simulink model "button"  (R2021b)
settings: Solver=FixedStepDiscrete  StartTime=0.0  StopTime=inf  FixedStep=0.01  RelTol=1e-3
libraries: robotlib x11, simulink x2
settings Model: Creator=alessandrini  LastModifiedBy=alessandrini
settings OptimizationCC: EnhancedBackFolding=on  PassReuseOutputArgsAs=Individual arguments  ZeroExternalMemoryAtStartup=off  ZeroInternalMemoryAtStartup=off  MaxStackSize=64  OptimizeBlockOrder=speed  DifferentSizesBufferReuse=on  OptimizationCustomize=off  EfficientTunableParamExpr=on
settings DebuggingCC: ParameterTunabilityLossMsg=error
settings HardwareCC: ProdBitPerPointer=32  ProdBitPerSizeT=32  ProdBitPerPtrDiffT=32  ProdLargestAtomicFloat=None  ProdIntDivRoundTo=Undefined  ProdEndianess=Unspecified  ProdWordSize=32  ProdHWDeviceType=Generic->Unspecified (assume 32-bit Generic)  UseEmbeddedCoderFeatures=off
settings RTWCC: Description=Embedded Coder  SystemTargetFile=ert.tlc  HardwareBoard=Robot Operating System (ROS)  TLCOptions="-aInlineSetEventsForThisBaseRateFcn=TLC_FALSE -aSuppressMultiTaskScheduler=TLC_FALSE  -aRateBasedStepFcn=0"  TemplateMakefile=ert_default_tmf  Toolchain=Catkin  TargetLang=C++
settings CodeAppCC: ForceParamTrailComments=on  IgnoreCustomStorageClasses=off  OperatorAnnotations=on  SimulinkDataObjDesc=on  SFDataObjDesc=on  InsertBlockDesc=on
settings ERTTargetCC: SupportNonInlinedSFcns=on

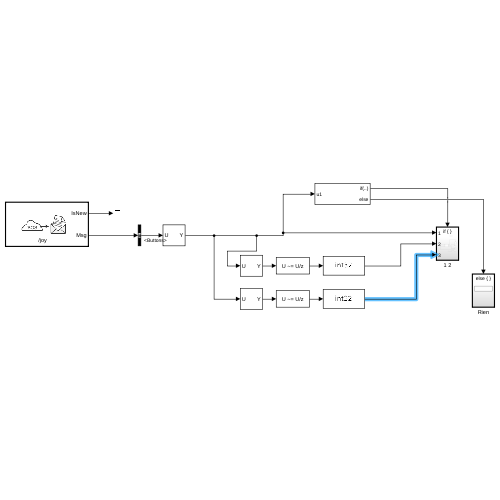
[thumbnail: Simulink's stored preview of the top-level diagram]
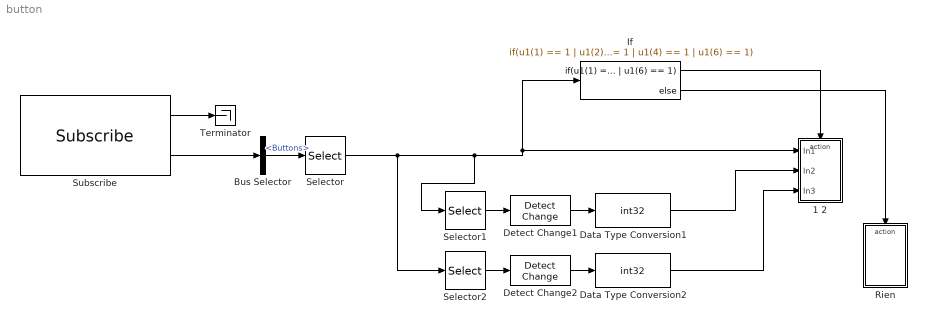
== system button ==
  1 2 : Subsystem
  Bus Selector : BusSelector  OutputSignals=Buttons
  Data Type Conversion1 : DataTypeConversion  OutDataTypeStr=int32
  Data Type Conversion2 : DataTypeConversion  OutDataTypeStr=int32
  Detect Change1 : simulink/Logic and Bit Operations/Detect Change  vinit=0  OutDataTypeStr=boolean
  Detect Change2 : simulink/Logic and Bit Operations/Detect Change  vinit=0  OutDataTypeStr=boolean
  If : If  IfExpression=u1(1) == 1 | u1(2) == 1 | u1(3) == 1 | u1(4) == 1 | u1(6) == 1
  Rien : Subsystem
  Selector : Selector  InputPortWidth=128  IndexOptions=Index vector (dialog)  Indices=[1 2 3 4 5 6]  OutputSizes=1
  Selector1 : Selector  InputPortWidth=6  IndexOptions=Index vector (dialog)  Indices=[1]  OutputSizes=1
  Selector2 : Selector  InputPortWidth=6  IndexOptions=Index vector (dialog)  Indices=[3]  OutputSizes=1
  Subscribe : robotlib/Subscribe  topicSource=Select from ROS network  topic=/joy  messageType=sensor_msgs/Joy  SampleTime=-1  legacyBusStruct=off  messageQueueLength=1
  Terminator : Terminator
  wires:
  Subscribe/2 -> Bus Selector/1
  Subscribe/1 -> Terminator/1
  If/2 -> Rien/Action
  If/1 -> 1 2/Action
  Bus Selector/1 -> Selector/1  "<Buttons>"
  Selector/1 -> Selector2/1, Selector1/1, If/1, 1 2/1(In1)
  Detect Change1/1 -> Data Type Conversion1/1
  Data Type Conversion1/1 -> 1 2/2(In2)
  Selector1/1 -> Detect Change1/1
  Selector2/1 -> Detect Change2/1
  Detect Change2/1 -> Data Type Conversion2/1
  Data Type Conversion2/1 -> 1 2/3(In3)

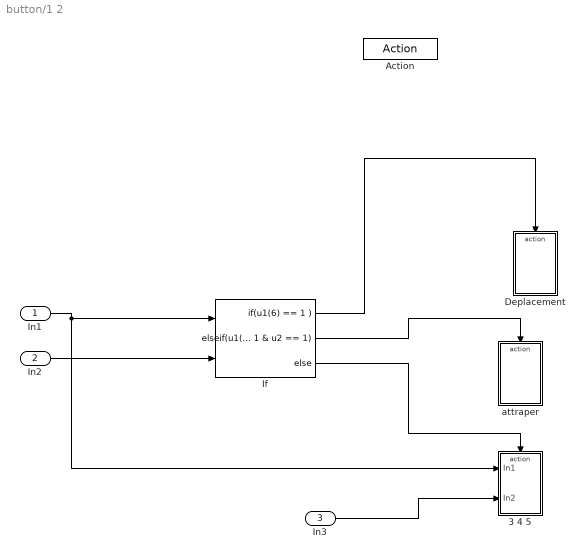
== system button/1 2 ==
  In1 : Inport
  In2 : Inport  Port=2
  In3 : Inport  Port=3
  Action : ActionPort  InitializeStates=reset  ActionPortLabel=if(u1(1) == 1 | u1(2) == 1 | u1(3) == 1 | u1(4) == 1 | u1(6) == 1)
  3 4 5 : Subsystem
  Deplacement : Subsystem
  If : If  NumInputs=2  IfExpression=u1(6) == 1  ElseIfExpressions=u1(1) == 1 & u2 == 1
  attraper : Subsystem
  wires:
  In1/1 -> 3 4 5/1(In1), If/1
  If/1 -> Deplacement/Action
  If/2 -> attraper/Action
  If/3 -> 3 4 5/Action
  In2/1 -> If/2
  In3/1 -> 3 4 5/2(In2)

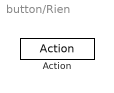
== system button/Rien ==
  Action : ActionPort  InitializeStates=reset  ActionPortLabel=else

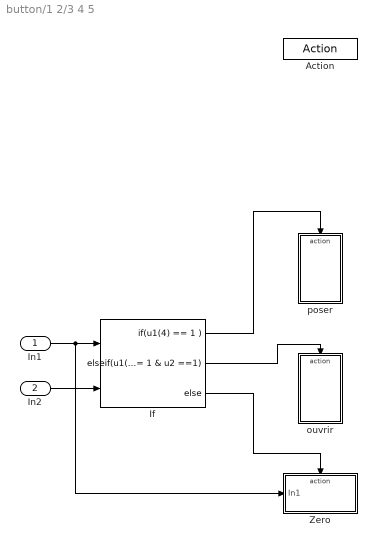
== system button/1 2/3 4 5 ==
  In1 : Inport
  In2 : Inport  Port=2
  Action : ActionPort  InitializeStates=reset  ActionPortLabel=else
  If : If  NumInputs=2  IfExpression=u1(4) == 1  ElseIfExpressions=u1(3) == 1 & u2 ==1
  "Zero " : Subsystem  TreatAsAtomicUnit=on
  ouvrir : Subsystem
  poser : Subsystem
  wires:
  If/3 -> "Zero "/Action
  If/2 -> ouvrir/Action
  In1/1 -> "Zero "/1(In1), If/1
  If/1 -> poser/Action
  In2/1 -> If/2

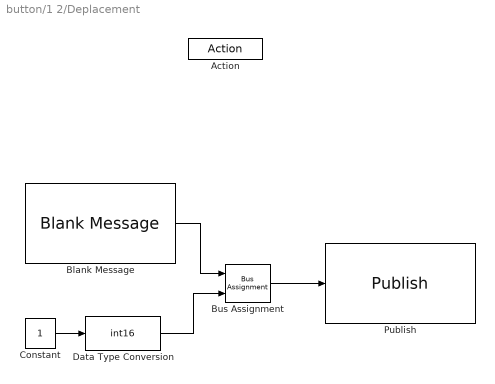
== system button/1 2/Deplacement ==
  Action : ActionPort  InitializeStates=reset  ActionPortLabel=if(u1(6) == 1 )
  Blank Message : robotlib/Blank Message  messageClass=Message  entityType=std_msgs/Int16  messageType=std_msgs/Int16  SampleTime=inf  legacyBusStruct=off
  Bus Assignment : BusAssignment  AssignedSignals=Data
  Constant : Constant
  Data Type Conversion : DataTypeConversion  OutDataTypeStr=int16
  Publish : robotlib/Publish  topicSource=Specify your own  topic=/etat  messageType=std_msgs/Int16  legacyBusStruct=off  messageQueueLength=1
  wires:
  Blank Message/1 -> Bus Assignment/1
  Bus Assignment/1 -> Publish/1
  Constant/1 -> Data Type Conversion/1
  Data Type Conversion/1 -> Bus Assignment/2
  ? -> ?
  ? -> ?

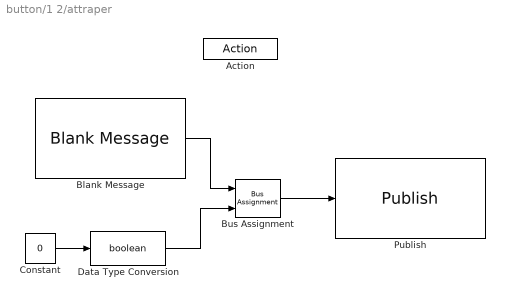
== system button/1 2/attraper ==
  Action : ActionPort  InitializeStates=reset  ActionPortLabel=elseif(u1(1) == 1 )
  Blank Message : robotlib/Blank Message  messageClass=Message  entityType=std_msgs/Bool  messageType=std_msgs/Bool  SampleTime=inf  legacyBusStruct=off
  Bus Assignment : BusAssignment  AssignedSignals=Data
  Constant : Constant  Value=0
  Data Type Conversion : DataTypeConversion  OutDataTypeStr=boolean
  Publish : robotlib/Publish  topicSource=Specify your own  topic=/hand  messageType=std_msgs/Bool  legacyBusStruct=off  messageQueueLength=1
  wires:
  Data Type Conversion/1 -> Bus Assignment/2
  Bus Assignment/1 -> Publish/1
  Constant/1 -> Data Type Conversion/1
  Blank Message/1 -> Bus Assignment/1

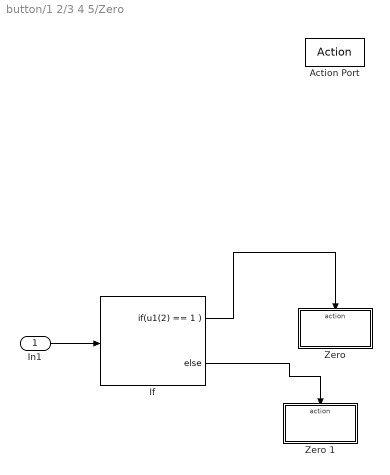
== system button/1 2/3 4 5/Zero  ==
  In1 : Inport
  Action Port : ActionPort  ActionPortLabel=else
  If : If  IfExpression=u1(2) == 1
  "Zero " : Subsystem  TreatAsAtomicUnit=on
  Zero 1 : Subsystem  TreatAsAtomicUnit=on
  wires:
  In1/1 -> If/1
  If/1 -> "Zero "/Action
  If/2 -> Zero 1/Action

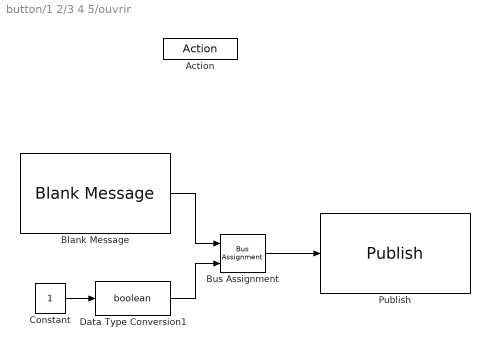
== system button/1 2/3 4 5/ouvrir ==
  Action : ActionPort  InitializeStates=reset  ActionPortLabel=elseif(u1(3) == 1 )
  Blank Message : robotlib/Blank Message  messageClass=Message  entityType=std_msgs/Bool  messageType=std_msgs/Bool  SampleTime=inf  legacyBusStruct=off
  Bus Assignment : BusAssignment  AssignedSignals=Data
  Constant : Constant
  Data Type Conversion1 : DataTypeConversion  OutDataTypeStr=boolean
  Publish : robotlib/Publish  topicSource=Specify your own  topic=/hand  messageType=std_msgs/Bool  legacyBusStruct=off  messageQueueLength=1
  wires:
  Data Type Conversion1/1 -> Bus Assignment/2
  Blank Message/1 -> Bus Assignment/1
  Constant/1 -> Data Type Conversion1/1
  Bus Assignment/1 -> Publish/1

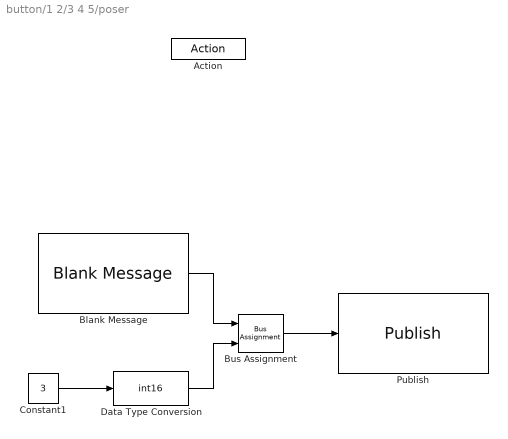
== system button/1 2/3 4 5/poser ==
  Action : ActionPort  InitializeStates=reset  ActionPortLabel=if(u1(4) == 1 )
  Blank Message : robotlib/Blank Message  messageClass=Message  entityType=std_msgs/Int16  messageType=std_msgs/Int16  SampleTime=inf  legacyBusStruct=off
  Bus Assignment : BusAssignment  AssignedSignals=Data
  Constant1 : Constant  Value=3
  Data Type Conversion : DataTypeConversion  OutDataTypeStr=int16
  Publish : robotlib/Publish  topicSource=Specify your own  topic=/etat  messageType=std_msgs/Int16  legacyBusStruct=off  messageQueueLength=1
  wires:
  Constant1/1 -> Data Type Conversion/1
  Blank Message/1 -> Bus Assignment/1
  Bus Assignment/1 -> Publish/1
  Data Type Conversion/1 -> Bus Assignment/2

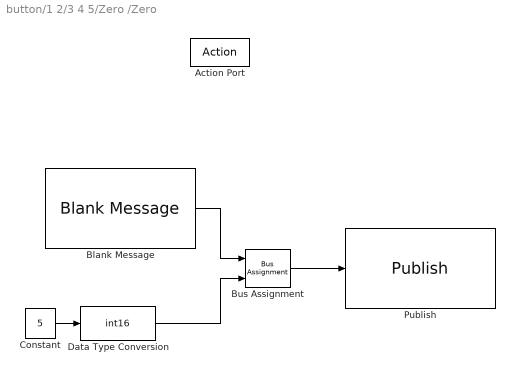
== system button/1 2/3 4 5/Zero /Zero  ==
  Action Port : ActionPort  ActionPortLabel=if(u1(4) == 1 )
  Blank Message : robotlib/Blank Message  messageClass=Message  entityType=std_msgs/Int16  messageType=std_msgs/Int16  SampleTime=inf  legacyBusStruct=off
  Bus Assignment : BusAssignment  AssignedSignals=Data
  Constant : Constant  Value=5
  Data Type Conversion : DataTypeConversion  OutDataTypeStr=int16
  Publish : robotlib/Publish  topicSource=Specify your own  topic=/etat  messageType=std_msgs/Int16  legacyBusStruct=off  messageQueueLength=1
  wires:
  Constant/1 -> Data Type Conversion/1
  Blank Message/1 -> Bus Assignment/1
  Bus Assignment/1 -> Publish/1
  Data Type Conversion/1 -> Bus Assignment/2

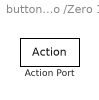
== system button/1 2/3 4 5/Zero /Zero 1 ==
  Action Port : ActionPort  ActionPortLabel=else
